simulink model "more_advanced"  (R2021a)
settings: Solver=VariableStepAuto  StartTime=0.0  StopTime=10.0  RelTol=1e-3
settings Model: Creator=matteopenlington  LastModifiedBy=matteopenlington

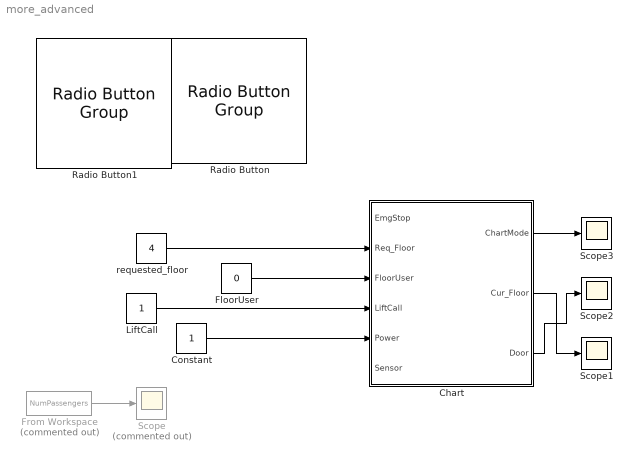
== system more_advanced ==
  Chart : Stateflow chart  TreatAsAtomicUnit=on
  Constant : Constant
  FloorUser : Constant  Value=0
  From Workspace : FromWorkspace  Commented=on  VariableName=NumPassengers  OutDataTypeStr=single  Interpolate=off  ZeroCross=off  OutputAfterFinalValue=Holding final value
  LiftCall : Constant
  Radio Button : RadioButtonGroup  SelectedLabel=0  ButtonGroupName=Group
      settings: Values={{'0', '1', '2', '3', '4', '5'}, [0 1 2 3 4 5]}
  Radio Button1 : RadioButtonGroup  SelectedLabel=4  ButtonGroupName=Group
      settings: Values={{'0', '1', '2', '3', '4', '5'}, [0 1 2 3 4 5]}
  Scope : Scope  Commented=on
  Scope1 : Scope
  Scope2 : Scope
  Scope3 : Scope
  requested_floor : Constant  Value=4
  wires:
  Constant/1 -> Chart/5(Power)
  Chart/3(Door) -> Scope2/1
  Chart/1(ChartMode) -> Scope3/1
  LiftCall/1 -> Chart/4(LiftCall)
  requested_floor/1 -> Chart/2(Req_Floor)
  Chart/2(Cur_Floor) -> Scope1/1
  From Workspace/1 -> Scope/1
  FloorUser/1 -> Chart/3(FloorUser)

== stateflow chart more_advanced/Chart ==
  state Initial
    entry:
    Cur_Floor = 0;
  note: This is for:
      | - lift is at floor 0.
      | - user calls lift from floor 0
      | - lift requested to floor 2
  state Idle_waiting
  state Go to floor
  state Idle_doors
    entry:
    exit:
    state DoorOpen
      entry:
      Door = 1;
    state DoorClose
      exit:
      Door = 0;
    (default) -> DoorOpen
    DoorClose -> DoorOpen [order 1] : [Door == 0 || Sensor == 1]
    DoorOpen -> DoorClose : [Door == 1]
    DoorClose -> Idle_doors [order 2] : [Door == 0 && Sensor == 0]
  state MovingUp
    entry:
    %Motor == 1;
    exit:
    %Motor == 0;
  state MovingDown
    entry:
    %Motor == -1;
    exit:
    %Motor == 0;
  (default) -> Initial
  Initial -> (junction 55)
  (junction 55) -> Idle_waiting [order 2] : [LiftCall ~= 1]
  (junction 55) -> (junction 66) [order 1] : [LiftCall == 1]
  (junction 66) -> (junction 67) : [Cur_Floor == FloorUser]
  (junction 67) -> Idle_doors
  Idle_doors -> MovingUp [order 1] : [Req_Floor > Cur_Floor]
  MovingUp -> Idle_doors : after(2,sec){Cur_Floor = Cur_Floor + 1}
  Idle_doors -> MovingDown [order 2] : [Req_Floor > Cur_Floor]
  MovingDown -> Idle_doors : after(2,sec){Cur_Floor = Cur_Floor - 1}
  data: ChartMode output Enum: ChartModeType; EmgStop input; Req_Floor input; FloorUser input; LiftCall input; Power input; Sensor input; Cur_Floor output double; Door output
